simulink model "gate_V26_2016a"  (R2016a)
settings: Solver=FixedStepDiscrete  StartTime=0.0  StopTime=100  FixedStep=0.001  RelTol=1e-3
undefined symbols (not defined in the file or in its folder): CLOSE_CHAR, CLOSE_SIDE_VALUE, CLOSED, CLOSING, NO_PASS_ASSIG, OPEN, OPEN_CHAR, OPEN_SIDE_VALUE, OPEN_TIMEOUT, OPENING, OPENING_ACTIVE, PASS_ASSIGNED, PASS_INCOMPLETE, PASS_TIMEOUT, PASSWORD_VERIFIED, sigbuilder_block, TIMEOUT, WRONG_PASSWORD
libraries: simulink x9, arduinolib x5
(part 1 of 3)
settings Model: ExtModeTrigDuration=2  Creator=omaro  LastModifiedBy=omaro
settings OptimizationCC: StateBitsets=on  DataBitsets=on  LifeSpan=1  MaxStackSize=64
settings DebuggingCC: ConsistencyChecking=error  ArrayBoundsChecking=error  SignalInfNanChecking=error  SignalRangeChecking=error  ReadBeforeWriteMsg=EnableAllAsError  WriteAfterWriteMsg=EnableAllAsError  WriteAfterReadMsg=EnableAllAsError  AlgebraicLoopMsg=error  ArtificialAlgebraicLoopMsg=error  BlockPriorityViolationMsg=error  MinStepSizeMsg=error  CheckMatrixSingularityMsg=error  ParameterUnderflowMsg=error  ParameterPrecisionLossMsg=error  UnderSpecifiedDataTypeMsg=warning  UnnecessaryDatatypeConvMsg=warning  VectorMatrixConversionMsg=error  SignalLabelMismatchMsg=error  UnconnectedInputMsg=error  UnconnectedOutputMsg=error  UnconnectedLineMsg=error  SFcnCompatibilityMsg=warning  UniqueDataStoreMsg=error  BusObjectLabelMismatch=error  RootOutportRequireBusObject=error  ModelReferenceIOMsg=error  ModelReferenceVersionMismatchMessage=error  ModelReferenceIOMismatchMessage=error  ModelReferenceDataLoggingMessage=error  StrictBusMsg=ErrorOnBusTreatedAsVector  SFUnusedDataAndEventsDiag=error  SFUnexpectedBacktrackingDiag=error  SFInvalidInputDataAccessInChartInitDiag=error  SFNoUnconditionalDefaultTransitionDiag=error  SFTransitionOutsideNaturalParentDiag=error  SFUndirectedBroadcastEventsDiag=error  SFTransitionActionBeforeConditionDiag=error  SFOutputUsedAsStateInMooreChartDiag=warning
settings HardwareCC: ProdBitPerInt=16  ProdBitPerPointer=16  ProdLargestAtomicFloat=None  ProdWordSize=8  ProdHWDeviceType=Atmel->AVR
settings SFSimCC: SimCustomHeaderCode=|
  | //#include "C:\Users\omaro\Desktop\Gate_Model\Arduino\Arduino.h"
  | //#include "Keypad\Keypad.h"
settings RTWCC: SystemTargetFile=ert.tlc  HardwareBoard=Arduino Nano 3.0  TemplateMakefile=ert_default_tmf  GenerateReport=on  RTWUseSimCustomCode=on  Toolchain=Arduino AVR v1.6.1  BuildConfiguration=Faster Runs  LaunchReport=on
settings RTWCC: CustomHeaderCode=|
  | //#include "C:\Users\omaro\Desktop\Gate_Model\Arduino\Arduino.h"
  | //#include "Keypad\Keypad.h"
settings CodeAppCC: ForceParamTrailComments=on  OperatorAnnotations=on  MATLABSourceComments=on
settings ERTTargetCC: ERTCustomFileBanners=off  SupportContinuousTime=on  SupportNonInlinedSFcns=on  SupportVariableSizeSignals=on  ModelStepFunctionPrototypeControlCompliant=off  RootIOFormat=Structure reference

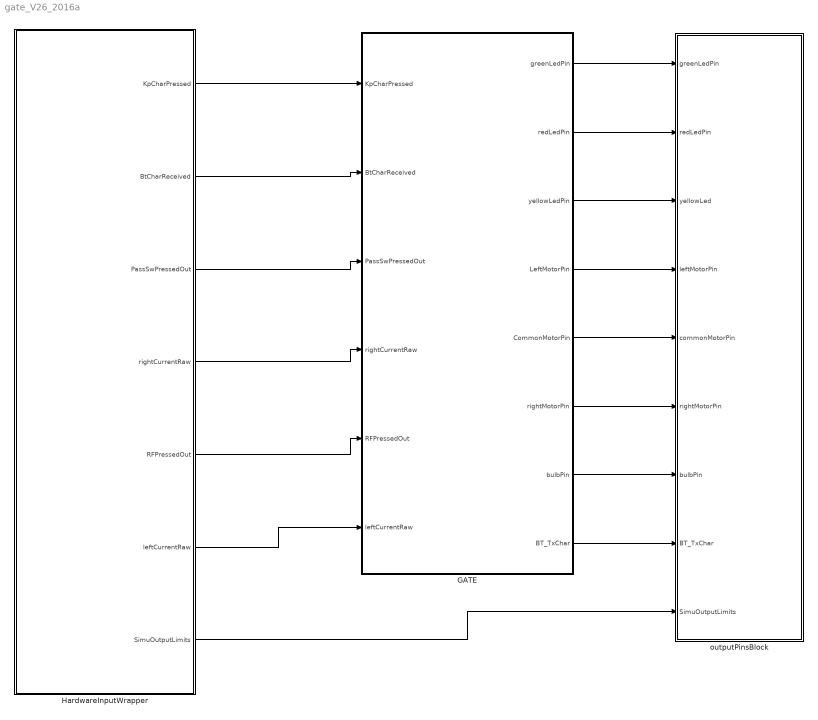
== system gate_V26_2016a ==
  GATE : Subsystem  Variant=on  VariantControl=Variant1  OverrideUsingVariant=Variant2
  HardwareInputWrapper : Subsystem  Variant=on  VariantControl=Variant1  OverrideUsingVariant=Variant2
  outputPinsBlock : Subsystem  Variant=on  VariantControl=Variant1  OverrideUsingVariant=Variant
  wires:
  HardwareInputWrapper/7(SimuOutputLimits) -> outputPinsBlock/9(SimuOutputLimits)
  HardwareInputWrapper/1(KpCharPressed) -> GATE/1("KpCharPressed ")
  HardwareInputWrapper/2(BtCharReceived) -> GATE/2("BtCharReceived ")
  HardwareInputWrapper/3(PassSwPressedOut) -> GATE/3("PassSwPressedOut ")
  HardwareInputWrapper/4(rightCurrentRaw) -> GATE/4(rightCurrentRaw)
  HardwareInputWrapper/5(RFPressedOut) -> GATE/5("RFPressedOut ")
  GATE/1(" greenLedPin") -> outputPinsBlock/1(greenLedPin)
  GATE/2(" redLedPin") -> outputPinsBlock/2(redLedPin)
  GATE/3(" yellowLedPin") -> outputPinsBlock/3(yellowLed)
  GATE/4(" LeftMotorPin") -> outputPinsBlock/4(leftMotorPin)
  GATE/5(" CommonMotorPin") -> outputPinsBlock/5(commonMotorPin)
  GATE/6(" rightMotorPin") -> outputPinsBlock/6(rightMotorPin)
  GATE/7(" bulbPin") -> outputPinsBlock/7(bulbPin)
  GATE/8(" BT_TxChar") -> outputPinsBlock/8(BT_TxChar)
  HardwareInputWrapper/6(leftCurrentRaw) -> GATE/6(leftCurrentRaw)

== system gate_V26_2016a/GATE ==
  "KpCharPressed " : Inport
  "BtCharReceived " : Inport  Port=2
  "PassSwPressedOut " : Inport  Port=3
  rightCurrentRaw : Inport  Port=4
  "RFPressedOut " : Inport  Port=5
  leftCurrentRaw : Inport  Port=6
  GATE_A : Subsystem  VariantControl=Variant1
  GATE_B : Subsystem  VariantControl=Variant2
  GATE_C : Subsystem  VariantControl=Variant3
  " greenLedPin" : Outport
  " redLedPin" : Outport  Port=2
  " yellowLedPin" : Outport  Port=3
  " LeftMotorPin" : Outport  Port=4
  " CommonMotorPin" : Outport  Port=5
  " rightMotorPin" : Outport  Port=6
  " bulbPin" : Outport  Port=7
  " BT_TxChar" : Outport  Port=8

== system gate_V26_2016a/HardwareInputWrapper ==
  HIL : Subsystem  VariantControl=Variant2
  MIL : Subsystem  VariantControl=Variant
  KpCharPressed : Outport
  BtCharReceived : Outport  Port=2
  PassSwPressedOut : Outport  Port=3
  rightCurrentRaw : Outport  Port=4
  RFPressedOut : Outport  Port=5
  leftCurrentRaw : Outport  Port=6
  SimuOutputLimits : Outport  Port=7

== system gate_V26_2016a/outputPinsBlock ==
  greenLedPin : Inport
  redLedPin : Inport  Port=2
  yellowLed : Inport  Port=3
  leftMotorPin : Inport  Port=4
  commonMotorPin : Inport  Port=5
  rightMotorPin : Inport  Port=6
  bulbPin : Inport  Port=7
  BT_TxChar : Inport  Port=8
  SimuOutputLimits : Inport  Port=9
  HIL : Subsystem  VariantControl=Variant
  MIL : Subsystem  Variant=on  VariantControl=Variant1  OverrideUsingVariant=Variant1

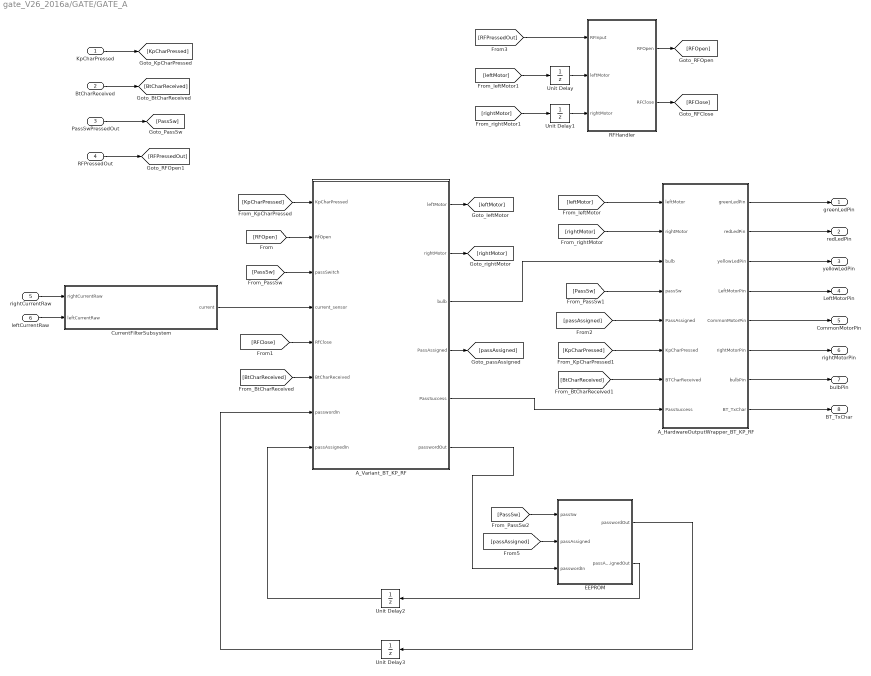
== system gate_V26_2016a/GATE/GATE_A ==
  KpCharPressed : Inport
  BtCharReceived : Inport  Port=2
  PassSwPressedOut : Inport  Port=3
  RFPressedOut : Inport  Port=4
  rightCurrentRaw : Inport  Port=5
  leftCurrentRaw : Inport  Port=6
  A_HardwareOutputWrapper_BT_KP_RF : Subsystem  VariantControl=Variant1
  A_Variant_BT_KP_RF : Subsystem  VariantControl=Variant
  CurrentFilterSubsystem : Subsystem
  EEPROM : Subsystem
  RFHandler : Subsystem
  Unit Delay{,1..3} (4 alike) : UnitDelay  SampleTime=-1
  greenLedPin : Outport
  redLedPin : Outport  Port=2
  yellowLedPin : Outport  Port=3
  LeftMotorPin : Outport  Port=4
  CommonMotorPin : Outport  Port=5
  rightMotorPin : Outport  Port=6
  bulbPin : Outport  Port=7
  BT_TxChar : Outport  Port=8
  wires:
  RFHandler/1(RFOpen) -> [RFOpen]
  RFHandler/2(RFClose) -> [RFClose]
  [RFPressedOut] -> RFHandler/1(RFInput)
  RFPressedOut/1 -> [RFPressedOut]
  PassSwPressedOut/1 -> [PassSw]
  [leftMotor] -> Unit Delay/1
  Unit Delay/1 -> RFHandler/2(leftMotor)
  [rightMotor] -> Unit Delay1/1
  Unit Delay1/1 -> RFHandler/3(rightMotor)
  BtCharReceived/1 -> [BtCharReceived]
  KpCharPressed/1 -> [KpCharPressed]
  [RFOpen] -> A_Variant_BT_KP_RF/2(RfOpen)
  [PassSw] -> A_Variant_BT_KP_RF/3(passSwitch)
  [RFClose] -> A_Variant_BT_KP_RF/5(RfClose)
  [BtCharReceived] -> A_Variant_BT_KP_RF/6(BtCharReceived)
  A_Variant_BT_KP_RF/1(leftMotor) -> [leftMotor]
  A_Variant_BT_KP_RF/2(rightMotor) -> [rightMotor]
  [KpCharPressed] -> A_Variant_BT_KP_RF/1(KpCharPressed)
  [leftMotor] -> A_HardwareOutputWrapper_BT_KP_RF/1(leftMotor)
  [rightMotor] -> A_HardwareOutputWrapper_BT_KP_RF/2(rightMotor)
  A_Variant_BT_KP_RF/3(bulb) -> A_HardwareOutputWrapper_BT_KP_RF/3(bulb)
  [PassSw] -> A_HardwareOutputWrapper_BT_KP_RF/4(passSw)
  [KpCharPressed] -> A_HardwareOutputWrapper_BT_KP_RF/6(KpCharPressed)
  [BtCharReceived] -> A_HardwareOutputWrapper_BT_KP_RF/7(BTCharReceived)
  A_HardwareOutputWrapper_BT_KP_RF/1(greenLedPin) -> greenLedPin/1
  A_HardwareOutputWrapper_BT_KP_RF/2(redLedPin) -> redLedPin/1
  A_HardwareOutputWrapper_BT_KP_RF/3(yellowLedPin) -> yellowLedPin/1
  A_HardwareOutputWrapper_BT_KP_RF/4(LeftMotorPin) -> LeftMotorPin/1
  A_HardwareOutputWrapper_BT_KP_RF/5(CommonMotorPin) -> CommonMotorPin/1
  A_HardwareOutputWrapper_BT_KP_RF/6(rightMotorPin) -> rightMotorPin/1
  A_HardwareOutputWrapper_BT_KP_RF/7(bulbPin) -> bulbPin/1
  A_HardwareOutputWrapper_BT_KP_RF/8(BT_TxChar) -> BT_TxChar/1
  A_Variant_BT_KP_RF/4(PassAssigned) -> [passAssigned]
  [passAssigned] -> A_HardwareOutputWrapper_BT_KP_RF/5(PassAssigned)
  [passAssigned] -> EEPROM/2(passAssigned)
  [PassSw] -> EEPROM/1(passSw)
  A_Variant_BT_KP_RF/6(passwordOut) -> EEPROM/3(passwordIn)
  EEPROM/1(passwordOut) -> Unit Delay3/1
  EEPROM/2(passAssignedOut) -> Unit Delay2/1
  Unit Delay2/1 -> A_Variant_BT_KP_RF/8(passAssignedIn)
  Unit Delay3/1 -> A_Variant_BT_KP_RF/7(passwordIn)
  A_Variant_BT_KP_RF/5(PassSuccess) -> A_HardwareOutputWrapper_BT_KP_RF/8(PassSuccess)
  CurrentFilterSubsystem/1(current) -> A_Variant_BT_KP_RF/4(current_sensor)
  rightCurrentRaw/1 -> CurrentFilterSubsystem/1(rightCurrentRaw)
  leftCurrentRaw/1 -> CurrentFilterSubsystem/2(leftCurrentRaw)

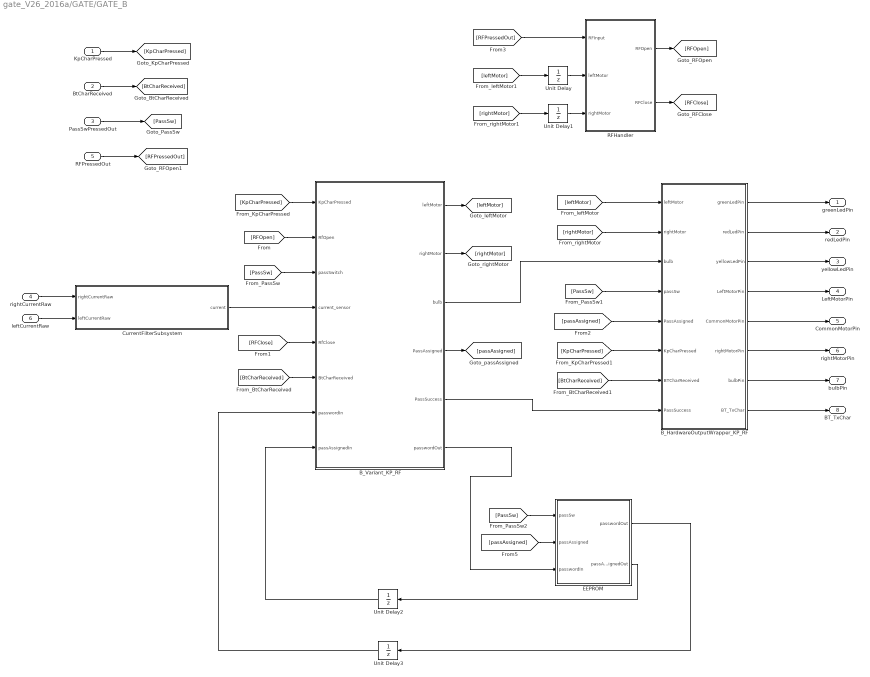
== system gate_V26_2016a/GATE/GATE_B ==
  KpCharPressed : Inport
  BtCharReceived : Inport  Port=2
  PassSwPressedOut : Inport  Port=3
  rightCurrentRaw : Inport  Port=4
  RFPressedOut : Inport  Port=5
  leftCurrentRaw : Inport  Port=6
  B_HardwareOutputWrapper_KP_RF : Subsystem  VariantControl=Variant2
  B_Variant_KP_RF : Subsystem  VariantControl=Variant2
  CurrentFilterSubsystem : Subsystem
  EEPROM : Subsystem
  RFHandler : Subsystem
  Unit Delay{,1..3} (4 alike) : UnitDelay  SampleTime=-1
  greenLedPin : Outport
  redLedPin : Outport  Port=2
  yellowLedPin : Outport  Port=3
  LeftMotorPin : Outport  Port=4
  CommonMotorPin : Outport  Port=5
  rightMotorPin : Outport  Port=6
  bulbPin : Outport  Port=7
  BT_TxChar : Outport  Port=8
  wires:
  CurrentFilterSubsystem/1(current) -> B_Variant_KP_RF/4(current_sensor)
  B_Variant_KP_RF/5(PassSuccess) -> B_HardwareOutputWrapper_KP_RF/8(PassSuccess)
  Unit Delay3/1 -> B_Variant_KP_RF/7(passwordIn)
  Unit Delay2/1 -> B_Variant_KP_RF/8(passAssignedIn)
  EEPROM/2(passAssignedOut) -> Unit Delay2/1
  EEPROM/1(passwordOut) -> Unit Delay3/1
  B_Variant_KP_RF/6(passwordOut) -> EEPROM/3(passwordIn)
  [PassSw] -> EEPROM/1(passSw)
  [passAssigned] -> EEPROM/2(passAssigned)
  [passAssigned] -> B_HardwareOutputWrapper_KP_RF/5(PassAssigned)
  B_Variant_KP_RF/4(PassAssigned) -> [passAssigned]
  B_HardwareOutputWrapper_KP_RF/8(BT_TxChar) -> BT_TxChar/1
  B_HardwareOutputWrapper_KP_RF/7(bulbPin) -> bulbPin/1
  B_HardwareOutputWrapper_KP_RF/6(rightMotorPin) -> rightMotorPin/1
  B_HardwareOutputWrapper_KP_RF/5(CommonMotorPin) -> CommonMotorPin/1
  B_HardwareOutputWrapper_KP_RF/4(LeftMotorPin) -> LeftMotorPin/1
  B_HardwareOutputWrapper_KP_RF/3(yellowLedPin) -> yellowLedPin/1
  B_HardwareOutputWrapper_KP_RF/2(redLedPin) -> redLedPin/1
  B_HardwareOutputWrapper_KP_RF/1(greenLedPin) -> greenLedPin/1
  [BtCharReceived] -> B_HardwareOutputWrapper_KP_RF/7(BTCharReceived)
  [KpCharPressed] -> B_HardwareOutputWrapper_KP_RF/6(KpCharPressed)
  [PassSw] -> B_HardwareOutputWrapper_KP_RF/4(passSw)
  B_Variant_KP_RF/3(bulb) -> B_HardwareOutputWrapper_KP_RF/3(bulb)
  [rightMotor] -> B_HardwareOutputWrapper_KP_RF/2(rightMotor)
  [leftMotor] -> B_HardwareOutputWrapper_KP_RF/1(leftMotor)
  [KpCharPressed] -> B_Variant_KP_RF/1(KpCharPressed)
  B_Variant_KP_RF/2(rightMotor) -> [rightMotor]
  B_Variant_KP_RF/1(leftMotor) -> [leftMotor]
  [BtCharReceived] -> B_Variant_KP_RF/6(BtCharReceived)
  [RFClose] -> B_Variant_KP_RF/5(RfClose)
  rightCurrentRaw/1 -> CurrentFilterSubsystem/1(rightCurrentRaw)
  [PassSw] -> B_Variant_KP_RF/3(passSwitch)
  [RFOpen] -> B_Variant_KP_RF/2(RfOpen)
  KpCharPressed/1 -> [KpCharPressed]
  BtCharReceived/1 -> [BtCharReceived]
  Unit Delay1/1 -> RFHandler/3(rightMotor)
  [rightMotor] -> Unit Delay1/1
  Unit Delay/1 -> RFHandler/2(leftMotor)
  [leftMotor] -> Unit Delay/1
  PassSwPressedOut/1 -> [PassSw]
  RFPressedOut/1 -> [RFPressedOut]
  [RFPressedOut] -> RFHandler/1(RFInput)
  RFHandler/2(RFClose) -> [RFClose]
  RFHandler/1(RFOpen) -> [RFOpen]
  leftCurrentRaw/1 -> CurrentFilterSubsystem/2(leftCurrentRaw)

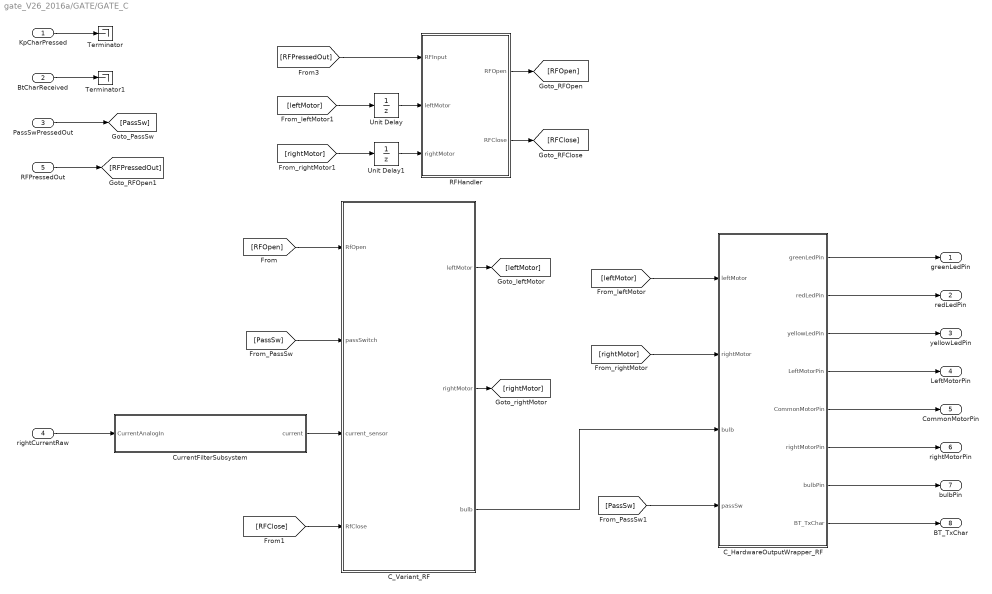
== system gate_V26_2016a/GATE/GATE_C ==
  KpCharPressed : Inport
  BtCharReceived : Inport  Port=2
  PassSwPressedOut : Inport  Port=3
  rightCurrentRaw : Inport  Port=4
  RFPressedOut : Inport  Port=5
  C_HardwareOutputWrapper_RF : Subsystem  VariantControl=Variant3
  C_Variant_RF : Subsystem  VariantControl=Variant3
  CurrentFilterSubsystem : Subsystem
  RFHandler : Subsystem
  Terminator : Terminator
  Terminator1 : Terminator
  Unit Delay : UnitDelay  SampleTime=-1
  Unit Delay1 : UnitDelay  SampleTime=-1
  greenLedPin : Outport
  redLedPin : Outport  Port=2
  yellowLedPin : Outport  Port=3
  LeftMotorPin : Outport  Port=4
  CommonMotorPin : Outport  Port=5
  rightMotorPin : Outport  Port=6
  bulbPin : Outport  Port=7
  BT_TxChar : Outport  Port=8
  wires:
  RFHandler/1(RFOpen) -> [RFOpen]
  RFHandler/2(RFClose) -> [RFClose]
  [RFPressedOut] -> RFHandler/1(RFInput)
  RFPressedOut/1 -> [RFPressedOut]
  PassSwPressedOut/1 -> [PassSw]
  [leftMotor] -> Unit Delay/1
  Unit Delay/1 -> RFHandler/2(leftMotor)
  [rightMotor] -> Unit Delay1/1
  Unit Delay1/1 -> RFHandler/3(rightMotor)
  BtCharReceived/1 -> Terminator1/1
  KpCharPressed/1 -> Terminator/1
  [RFOpen] -> C_Variant_RF/1(RfOpen)
  [PassSw] -> C_Variant_RF/2(passSwitch)
  rightCurrentRaw/1 -> CurrentFilterSubsystem/1(CurrentAnalogIn)
  [RFClose] -> C_Variant_RF/4(RfClose)
  C_Variant_RF/1(leftMotor) -> [leftMotor]
  C_Variant_RF/2(rightMotor) -> [rightMotor]
  [leftMotor] -> C_HardwareOutputWrapper_RF/1(leftMotor)
  [rightMotor] -> C_HardwareOutputWrapper_RF/2(rightMotor)
  C_Variant_RF/3(bulb) -> C_HardwareOutputWrapper_RF/3(bulb)
  [PassSw] -> C_HardwareOutputWrapper_RF/4(passSw)
  C_HardwareOutputWrapper_RF/1(greenLedPin) -> greenLedPin/1
  C_HardwareOutputWrapper_RF/2(redLedPin) -> redLedPin/1
  C_HardwareOutputWrapper_RF/3(yellowLedPin) -> yellowLedPin/1
  C_HardwareOutputWrapper_RF/4(LeftMotorPin) -> LeftMotorPin/1
  C_HardwareOutputWrapper_RF/5(CommonMotorPin) -> CommonMotorPin/1
  C_HardwareOutputWrapper_RF/6(rightMotorPin) -> rightMotorPin/1
  C_HardwareOutputWrapper_RF/7(bulbPin) -> bulbPin/1
  C_HardwareOutputWrapper_RF/8(BT_TxChar) -> BT_TxChar/1
  CurrentFilterSubsystem/1(current) -> C_Variant_RF/3(current_sensor)

== system gate_V26_2016a/HardwareInputWrapper/HIL ==
  Analog Input : arduinolib/Analog Input  pinNumber=6  sampleTime=-1  blockPlatform=arduino
  Analog Input1 : arduinolib/Analog Input  pinNumber=7  sampleTime=-1  blockPlatform=arduino
  BluetoothWrapper : Subsystem  Commented=on
  ButtonsPressed : Subsystem
  KeypadWrapper : Subsystem
  S-Function Builder1 : S-Function  Commented=on  InitFcn=try, set_param(gcb,'FunctionName','CurrentA_Lib'), end  FunctionName=CurrentA_Lib  SFunctionModules=CurrentA_Lib_wrapper  SFunctionDeploymentMode=off  EnableBusSupport=off  mask(S-Function Builder){}
      mask help: Simulink:masks:SFunctionBuilder_MD
      mask init:
      | val = [[.9  0.75 0.75 1 1 .9 .9 1]',[1 1 0.75 0.75 .9 .9 1 .9]'];try , sys = get_param(gcb,'SfunBuilderFcnName');if isempty(sys), sys = get_param(gcb,'FunctionName'); end,catch, sys = get_param(gcb,'FunctionName'); end
      settings: CopyFcn=set_param(gcbh,'LinkStatus','none')  PreSaveFcn=try, set_param(gcb,'FunctionName','CurrentA_Lib'), end  OpenFcn=sfunctionwizard(gcbh)
      mask Display: plot(val(:,1),val(:,2)),disp(sys), port_label('output',1,'currentValue')
  S-Function Builder2 : S-Function  Commented=on  InitFcn=try, set_param(gcb,'FunctionName','printingBlock'), end  FunctionName=printingBlock  SFunctionModules=printingBlock_wrapper  SFunctionDeploymentMode=off  EnableBusSupport=off  mask(S-Function Builder){}
      mask help: Simulink:masks:SFunctionBuilder_MD
      mask init: same as gate_V26_2016a/HardwareInputWrapper/HIL/S-Function Builder1
      settings: CopyFcn=set_param(gcbh,'LinkStatus','none')  PreSaveFcn=try, set_param(gcb,'FunctionName','printingBlock'), end  OpenFcn=sfunctionwizard(gcbh)
      mask Display: plot(val(:,1),val(:,2)),disp(sys), port_label('input',1,'uint8ToPrint')
  currentSensorWrapperOld : Subsystem  Commented=on
  KpCharPressed : Outport
  BtCharReceived : Outport  Port=2
  PassSwPressedOut : Outport  Port=3
  rightCurrentRaw : Outport  Port=4
  leftCurrentRaw : Outport  Port=5
  RFPressedOut : Outport  Port=6
  wires:
  BluetoothWrapper/1(bluetoothCharPressed) -> BtCharReceived/1
  Analog Input/1 -> rightCurrentRaw/1  "rightMotorSpeed"
  KeypadWrapper/1(charPressed) -> S-Function Builder2/1, KpCharPressed/1
  ButtonsPressed/2(SWPressed) -> PassSwPressedOut/1
  ButtonsPressed/1(RFPressed) -> RFPressedOut/1
  Analog Input1/1 -> leftCurrentRaw/1  "leftMotorSpeed"

== system gate_V26_2016a/HardwareInputWrapper/MIL ==
  Bus Creator : BusCreator  Inputs=16
  Quantizer{,1..3} (4 alike) : Quantizer  QuantizationInterval=-1
  Signal Builder : Subsystem  Tag=STV Subsys  LoadFcn=sigbuilder_block('load',[41.25 -234.75 971.25 378 ]);  StartFcn=sigbuilder_block('start');  StopFcn=sigbuilder_block('stop');  ClipboardFcn=sigbuilder_block('clipboard');  mask(Sigbuilder block){}
      mask help: Simulink:masks:SigbuilderBlock_MD
      mask init:
      | if ~strcmp(get_param(bdroot(gcbh),'SimulationStatus'),'stopped') tuvar = sigbuilder_block('maskInit'); end
      settings: CopyFcn=sigbuilder_block('copy');  DeleteFcn=sigbuilder_block('delete');  ModelCloseFcn=sigbuilder_block('modelClose');  PreSaveFcn=sigbuilder_block('preSave');  PauseFcn=sigbuilder_block('pause');  ContinueFcn=sigbuilder_block('continue');  NameChangeFcn=sigbuilder_block('namechange');  OpenFcn=sigbuilder_block('open',[6 28.2 1012.8 484.8 ]);  CloseFcn=sigbuilder_block('close');
      mask Display: plot(0, 0, 100, 100,[2, 2, 32, 32, 2], [68, 8, 8, 68, 68],[32, 2], [38, 38], [32, 19, 2],[53, 60, 44], [32, 17, 17, 2],[16, 16, 31, 31]);txt = getActiveGroup(gcbh);text(2, 100, txt,'verticalAlignment', 'top');
  KpCharPressed : Outport
  BtCharReceived : Outport  Port=2
  PassSwPressedOut : Outport  Port=3
  RFPressedOut : Outport  Port=4
  rightCurrentRaw : Outport  Port=5
  leftCurrentRaw : Outport  Port=6
  SimuOutputLimits : Outport  Port=7
  wires:
  Signal Builder/2(BT_input) -> Quantizer1/1
  Signal Builder/4(SW_input) -> Quantizer3/1
  Signal Builder/1(Kp_input) -> Quantizer/1
  Signal Builder/3(RF_input) -> Quantizer2/1
  Quantizer/1 -> KpCharPressed/1
  Quantizer1/1 -> BtCharReceived/1
  Quantizer2/1 -> RFPressedOut/1
  Quantizer3/1 -> PassSwPressedOut/1
  Bus Creator/1 -> SimuOutputLimits/1
  Signal Builder/17(GreenLedMax) -> Bus Creator/11  "GreenLedMax"
  Signal Builder/16(YellowLedMin) -> Bus Creator/10  "YellowLedMin"
  Signal Builder/18(GreenLedMin) -> Bus Creator/12  "GreenLedMin"
  Signal Builder/15(YellowLedMax) -> Bus Creator/9  "YellowLedMax"
  Signal Builder/19(BulbMax) -> Bus Creator/13  "BulbMax"
  Signal Builder/14(RedLedMin) -> Bus Creator/8  "RedLedMin"
  Signal Builder/20(BulbMin) -> Bus Creator/14  "BulbMin"
  Signal Builder/21(BT_outputMax) -> Bus Creator/15  "BT_outputMax"
  Signal Builder/13(RedLedMax) -> Bus Creator/7  "RedLedMax"
  Signal Builder/12(MCMin) -> Bus Creator/6  "MCMin"
  Signal Builder/11(MCMax) -> Bus Creator/5  "MCMax"
  Signal Builder/10(MRMin) -> Bus Creator/4  "MRMin"
  Signal Builder/9(MRMax) -> Bus Creator/3  "MRMax"
  Signal Builder/8(MLMin) -> Bus Creator/2  "MLMin"
  Signal Builder/7(MLMax) -> Bus Creator/1  "MLMax"
  Signal Builder/22(BT_outputMin) -> Bus Creator/16  "BT_outputMin"
  Signal Builder/5(rightSpeedRaw) -> rightCurrentRaw/1
  Signal Builder/6(leftSpeedRaw) -> leftCurrentRaw/1

== system gate_V26_2016a/outputPinsBlock/HIL ==
  greenLedPin : Inport
  redLedPin : Inport  Port=2
  yellowLed : Inport  Port=3
  leftMotorPin : Inport  Port=4
  commonMotorPin : Inport  Port=5
  rightMotorPin : Inport  Port=6
  bulbPin : Inport  Port=7
  Digital Output : arduinolib/Digital Output  pinNumber=11  blockPlatform=arduino
  Digital Output1 : arduinolib/Digital Output  pinNumber=12  blockPlatform=arduino
  Digital Output2 : arduinolib/Digital Output  pinNumber=13  blockPlatform=arduino
  S-Function Builder1 : S-Function  InitFcn=try, set_param(gcb,'FunctionName','A2PIN_Lib'), end  FunctionName=A2PIN_Lib  SFunctionModules=A2PIN_Lib_wrapper  SFunctionDeploymentMode=off  EnableBusSupport=off  mask(S-Function Builder){}
      mask help: Simulink:masks:SFunctionBuilder_MD
      mask init: same as gate_V26_2016a/HardwareInputWrapper/HIL/S-Function Builder1
      settings: CopyFcn=set_param(gcbh,'LinkStatus','none')  PreSaveFcn=try, set_param(gcb,'FunctionName','A2PIN_Lib'), end  OpenFcn=sfunctionwizard(gcbh)
      mask Display: plot(val(:,1),val(:,2)),disp(sys), port_label('input',1,'input')
  S-Function Builder2 : S-Function  InitFcn=try, set_param(gcb,'FunctionName','A3PIN_Lib'), end  FunctionName=A3PIN_Lib  SFunctionModules=A3PIN_Lib_wrapper  SFunctionDeploymentMode=off  EnableBusSupport=off  mask(S-Function Builder){}
      mask help: Simulink:masks:SFunctionBuilder_MD
      mask init: same as gate_V26_2016a/HardwareInputWrapper/HIL/S-Function Builder1
      settings: CopyFcn=set_param(gcbh,'LinkStatus','none')  PreSaveFcn=try, set_param(gcb,'FunctionName','A3PIN_Lib'), end  OpenFcn=sfunctionwizard(gcbh)
      mask Display: plot(val(:,1),val(:,2)),disp(sys), port_label('input',1,'input')
  S-Function Builder3 : S-Function  InitFcn=try, set_param(gcb,'FunctionName','A4PIN_Lib'), end  FunctionName=A4PIN_Lib  SFunctionModules=A4PIN_Lib_wrapper  SFunctionDeploymentMode=off  EnableBusSupport=off  mask(S-Function Builder){}
      mask help: Simulink:masks:SFunctionBuilder_MD
      mask init: same as gate_V26_2016a/HardwareInputWrapper/HIL/S-Function Builder1
      settings: CopyFcn=set_param(gcbh,'LinkStatus','none')  PreSaveFcn=try, set_param(gcb,'FunctionName','A4PIN_Lib'), end  OpenFcn=sfunctionwizard(gcbh)
      mask Display: plot(val(:,1),val(:,2)),disp(sys), port_label('input',1,'input')
  S-Function Builder4 : S-Function  InitFcn=try, set_param(gcb,'FunctionName','A5PIN_Lib'), end  FunctionName=A5PIN_Lib  SFunctionModules=A5PIN_Lib_wrapper  SFunctionDeploymentMode=off  EnableBusSupport=off  mask(S-Function Builder){}
      mask help: Simulink:masks:SFunctionBuilder_MD
      mask init: same as gate_V26_2016a/HardwareInputWrapper/HIL/S-Function Builder1
      settings: CopyFcn=set_param(gcbh,'LinkStatus','none')  PreSaveFcn=try, set_param(gcb,'FunctionName','A5PIN_Lib'), end  OpenFcn=sfunctionwizard(gcbh)
      mask Display: plot(val(:,1),val(:,2)),disp(sys), port_label('input',1,'input')
  wires:
  yellowLed/1 -> Digital Output2/1
  redLedPin/1 -> Digital Output/1
  greenLedPin/1 -> Digital Output1/1
  commonMotorPin/1 -> S-Function Builder3/1
  leftMotorPin/1 -> S-Function Builder2/1
  rightMotorPin/1 -> S-Function Builder4/1
  bulbPin/1 -> S-Function Builder1/1

== system gate_V26_2016a/outputPinsBlock/MIL ==
  "leftMotorPin " : Inport
  "commonMotorPin " : Inport  Port=2
  "rightMotorPin " : Inport  Port=3
  greenLedPin : Inport  Port=4
  redLedPin : Inport  Port=5
  yellowLed : Inport  Port=6
  bulbPin : Inport  Port=7
  BT_TxChar : Inport  Port=8
  SimuOutputLimits : Inport  Port=9
  ScopeBlocks : Subsystem  VariantControl=Variant1
  "VerificationBlocks " : Subsystem  VariantControl=Variant2

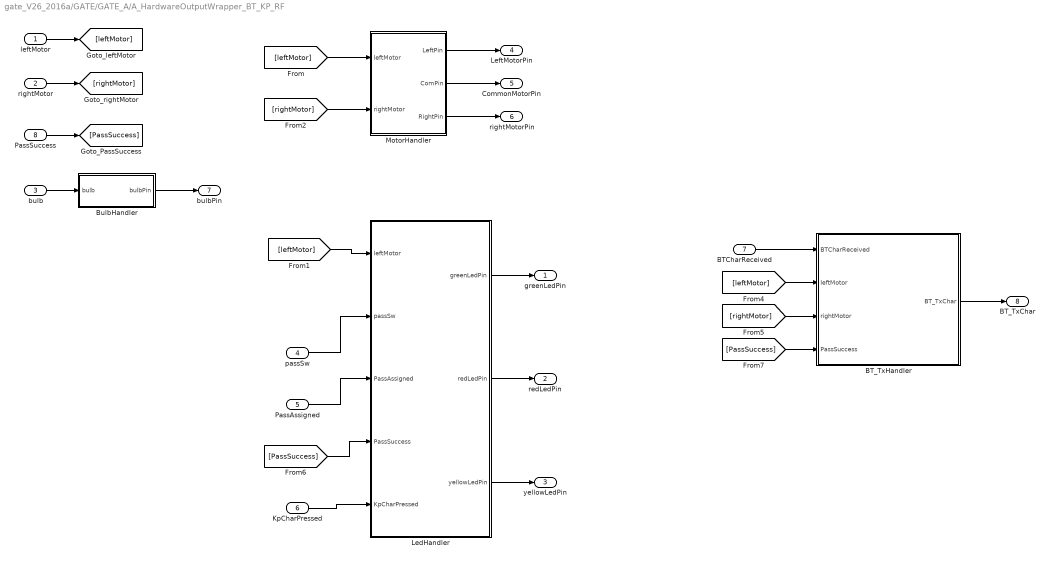
== system gate_V26_2016a/GATE/GATE_A/A_HardwareOutputWrapper_BT_KP_RF ==
  leftMotor : Inport
  rightMotor : Inport  Port=2
  bulb : Inport  Port=3
  passSw : Inport  Port=4
  PassAssigned : Inport  Port=5
  KpCharPressed : Inport  Port=6
  BTCharReceived : Inport  Port=7
  PassSuccess : Inport  Port=8
  BT_TxHandler : Subsystem
  BulbHandler : Subsystem
  LedHandler : Subsystem
  MotorHandler : Subsystem
  greenLedPin : Outport
  redLedPin : Outport  Port=2
  yellowLedPin : Outport  Port=3
  LeftMotorPin : Outport  Port=4
  CommonMotorPin : Outport  Port=5
  rightMotorPin : Outport  Port=6
  bulbPin : Outport  Port=7
  BT_TxChar : Outport  Port=8
  wires:
  [leftMotor] -> MotorHandler/1(leftMotor)
  [rightMotor] -> MotorHandler/2(rightMotor)
  bulb/1 -> BulbHandler/1(bulb)
  LedHandler/1(greenLedPin) -> greenLedPin/1
  LedHandler/2(redLedPin) -> redLedPin/1
  LedHandler/3(yellowLedPin) -> yellowLedPin/1
  MotorHandler/1(LeftPin) -> LeftMotorPin/1
  MotorHandler/2(ComPin) -> CommonMotorPin/1
  MotorHandler/3(RightPin) -> rightMotorPin/1
  BulbHandler/1(bulbPin) -> bulbPin/1
  leftMotor/1 -> [leftMotor]
  [leftMotor] -> LedHandler/1(leftMotor)
  rightMotor/1 -> [rightMotor]
  passSw/1 -> LedHandler/2(passSw)
  PassAssigned/1 -> LedHandler/3(PassAssigned)
  [PassSuccess] -> LedHandler/4(PassSuccess)
  KpCharPressed/1 -> LedHandler/5(KpCharPressed)
  [leftMotor] -> BT_TxHandler/2(leftMotor)
  BTCharReceived/1 -> BT_TxHandler/1(BTCharReceived)
  [rightMotor] -> BT_TxHandler/3(rightMotor)
  PassSuccess/1 -> [PassSuccess]
  [PassSuccess] -> BT_TxHandler/4(PassSuccess)
  BT_TxHandler/1(BT_TxChar) -> BT_TxChar/1

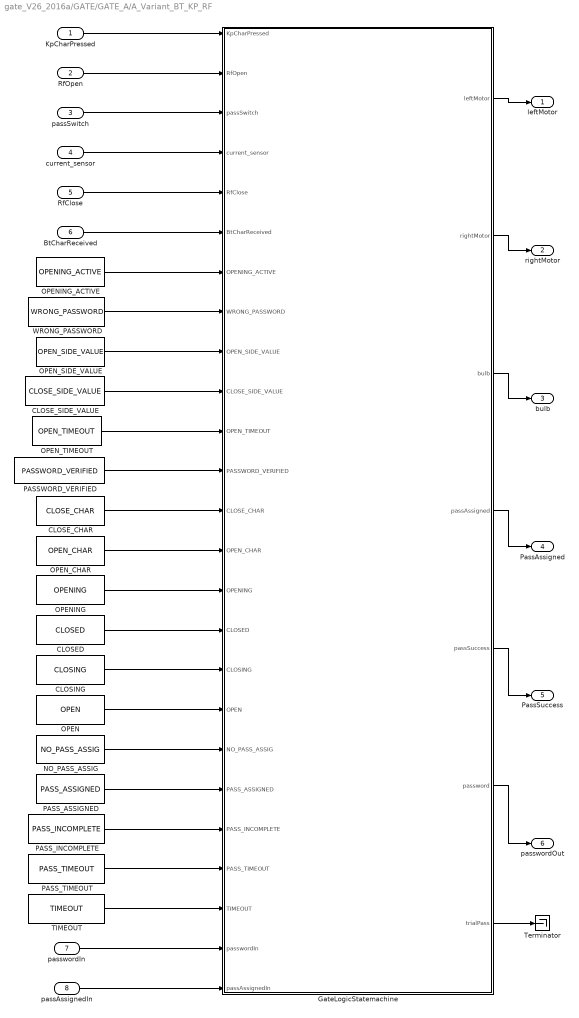
== system gate_V26_2016a/GATE/GATE_A/A_Variant_BT_KP_RF ==
  KpCharPressed : Inport
  RfOpen : Inport  Port=2
  passSwitch : Inport  Port=3
  current_sensor : Inport  Port=4
  RfClose : Inport  Port=5
  BtCharReceived : Inport  Port=6
  passwordIn : Inport  Port=7
  passAssignedIn : Inport  Port=8
  CLOSED : Constant  Value=CLOSED  SampleTime=-1
  CLOSE_CHAR : Constant  Value=CLOSE_CHAR  SampleTime=-1
  CLOSE_SIDE_VALUE : Constant  Value=CLOSE_SIDE_VALUE  SampleTime=-1
  CLOSING : Constant  Value=CLOSING  SampleTime=-1
  GateLogicStatemachine : Stateflow chart  TreatAsAtomicUnit=on
  NO_PASS_ASSIG : Constant  Value=NO_PASS_ASSIG  SampleTime=-1
  OPEN : Constant  Value=OPEN  SampleTime=-1
  OPENING : Constant  Value=OPENING  SampleTime=-1
  OPENING_ACTIVE : Constant  Value=OPENING_ACTIVE  SampleTime=-1
  OPEN_CHAR : Constant  Value=OPEN_CHAR  SampleTime=-1
  OPEN_SIDE_VALUE : Constant  Value=OPEN_SIDE_VALUE  SampleTime=-1
  OPEN_TIMEOUT : Constant  Value=OPEN_TIMEOUT  SampleTime=-1
  PASSWORD_VERIFIED : Constant  Value=PASSWORD_VERIFIED  SampleTime=-1
  PASS_ASSIGNED : Constant  Value=PASS_ASSIGNED  SampleTime=-1
  PASS_INCOMPLETE : Constant  Value=PASS_INCOMPLETE  SampleTime=-1
  PASS_TIMEOUT : Constant  Value=PASS_TIMEOUT  SampleTime=-1
  TIMEOUT : Constant  Value=TIMEOUT  SampleTime=-1
  Terminator : Terminator
  WRONG_PASSWORD : Constant  Value=WRONG_PASSWORD  SampleTime=-1
  leftMotor : Outport
  rightMotor : Outport  Port=2
  bulb : Outport  Port=3
  PassAssigned : Outport  Port=4
  PassSuccess : Outport  Port=5
  passwordOut : Outport  Port=6
  wires:
  RfClose/1 -> GateLogicStatemachine/5(RfClose)
  TIMEOUT/1 -> GateLogicStatemachine/23(TIMEOUT)
  PASS_INCOMPLETE/1 -> GateLogicStatemachine/21(PASS_INCOMPLETE)
  PASS_ASSIGNED/1 -> GateLogicStatemachine/20(PASS_ASSIGNED)
  GateLogicStatemachine/4(passAssigned) -> PassAssigned/1
  passSwitch/1 -> GateLogicStatemachine/3(passSwitch)
  GateLogicStatemachine/5(passSuccess) -> PassSuccess/1
  PASS_TIMEOUT/1 -> GateLogicStatemachine/22(PASS_TIMEOUT)
  KpCharPressed/1 -> GateLogicStatemachine/1(KpCharPressed)
  BtCharReceived/1 -> GateLogicStatemachine/6(BtCharReceived)
  NO_PASS_ASSIG/1 -> GateLogicStatemachine/19(NO_PASS_ASSIG)
  CLOSE_SIDE_VALUE/1 -> GateLogicStatemachine/10(CLOSE_SIDE_VALUE)
  OPEN_TIMEOUT/1 -> GateLogicStatemachine/11(OPEN_TIMEOUT)
  OPEN_SIDE_VALUE/1 -> GateLogicStatemachine/9(OPEN_SIDE_VALUE)
  OPENING_ACTIVE/1 -> GateLogicStatemachine/7(OPENING_ACTIVE)
  GateLogicStatemachine/2(rightMotor) -> rightMotor/1
  GateLogicStatemachine/1(leftMotor) -> leftMotor/1
  WRONG_PASSWORD/1 -> GateLogicStatemachine/8(WRONG_PASSWORD)
  current_sensor/1 -> GateLogicStatemachine/4(current_sensor)
  GateLogicStatemachine/3(bulb) -> bulb/1
  RfOpen/1 -> GateLogicStatemachine/2(RfOpen)
  PASSWORD_VERIFIED/1 -> GateLogicStatemachine/12(PASSWORD_VERIFIED)
  OPEN/1 -> GateLogicStatemachine/18(OPEN)
  CLOSE_CHAR/1 -> GateLogicStatemachine/13(CLOSE_CHAR)
  OPEN_CHAR/1 -> GateLogicStatemachine/14(OPEN_CHAR)
  CLOSED/1 -> GateLogicStatemachine/16(CLOSED)
  OPENING/1 -> GateLogicStatemachine/15(OPENING)
  CLOSING/1 -> GateLogicStatemachine/17(CLOSING)
  GateLogicStatemachine/6(password) -> passwordOut/1
  passwordIn/1 -> GateLogicStatemachine/24(passwordIn)
  passAssignedIn/1 -> GateLogicStatemachine/25(passAssignedIn)
  GateLogicStatemachine/7(trialPass) -> Terminator/1

== system gate_V26_2016a/GATE/GATE_A/CurrentFilterSubsystem ==
  rightCurrentRaw : Inport
  leftCurrentRaw : Inport  Port=2
  10msSmapler : Stateflow chart  TreatAsAtomicUnit=on
  Subsystem : Subsystem
  current : Outport
  wires:
  10msSmapler/1(triggerOn()) -> Subsystem/Trigger
  Subsystem/1(current) -> current/1
  rightCurrentRaw/1 -> Subsystem/1(rightCurrentRaw)
  leftCurrentRaw/1 -> Subsystem/2(leftCurrentRaw)

== system gate_V26_2016a/GATE/GATE_A/EEPROM ==
  passSw : Inport
  passAssigned : Inport  Port=2
  passwordIn : Inport  Port=3
  EEPROM_Control : Stateflow chart  TreatAsAtomicUnit=on
  EEPROM_UPDATE : Subsystem  TreatAsAtomicUnit=on
  Terminator : Terminator
  Unit Delay : UnitDelay  SampleTime=-1
  Unit Delay1 : UnitDelay  SampleTime=-1
  passwordOut : Outport
  passAssignedOut : Outport  Port=2
  wires:
  passSw/1 -> EEPROM_Control/1(passSw)
  Unit Delay/1 -> EEPROM_Control/3(readComplete)
  Unit Delay1/1 -> EEPROM_Control/4(writeComplete)
  EEPROM_Control/1(clearReq) -> EEPROM_UPDATE/1(clearReq)
  EEPROM_Control/2(readReq) -> EEPROM_UPDATE/2(readReq)
  EEPROM_Control/3(writeReq) -> EEPROM_UPDATE/3(writeReq)
  passwordIn/1 -> EEPROM_UPDATE/4(passwordIn)
  [passAssigned] -> EEPROM_Control/2(passAssigned)
  [passAssigned] -> EEPROM_UPDATE/5(passAssignedIn)
  passAssigned/1 -> [passAssigned]
  EEPROM_UPDATE/1(readComplete) -> [readComplete]
  [readComplete] -> Unit Delay/1
  [writeComplete] -> Unit Delay1/1
  EEPROM_UPDATE/2(writeComplete) -> [writeComplete]
  EEPROM_UPDATE/4(passwordOut) -> passwordOut/1
  EEPROM_UPDATE/5(passAssignedOut) -> passAssignedOut/1
  EEPROM_UPDATE/3(clearComplete) -> Terminator/1

== system gate_V26_2016a/GATE/GATE_A/RFHandler ==
  RFInput : Inport
  leftMotor : Inport  Port=2
  rightMotor : Inport  Port=3
  CLOSED : Constant  Value=CLOSED  SampleTime=-1
  CLOSING : Constant  Value=CLOSING  SampleTime=-1
  OPEN : Constant  Value=OPEN  SampleTime=-1
  OPENING : Constant  Value=OPENING  SampleTime=-1
  RFHandlerL : Stateflow chart  TreatAsAtomicUnit=on
  Scope : Scope
  RFOpen : Outport
  RFClose : Outport  Port=2
  wires:
  RFInput/1 -> RFHandlerL/1(btn)
  RFHandlerL/1(RFClose) -> RFClose/1
  RFHandlerL/2(RFOpen) -> Scope/1, RFOpen/1
  OPEN/1 -> RFHandlerL/6(OPEN)
  CLOSING/1 -> RFHandlerL/5(CLOSING)
  CLOSED/1 -> RFHandlerL/4(CLOSED)
  OPENING/1 -> RFHandlerL/7(OPENING)
  leftMotor/1 -> RFHandlerL/2(leftMotor)
  rightMotor/1 -> RFHandlerL/3(rightMotor)

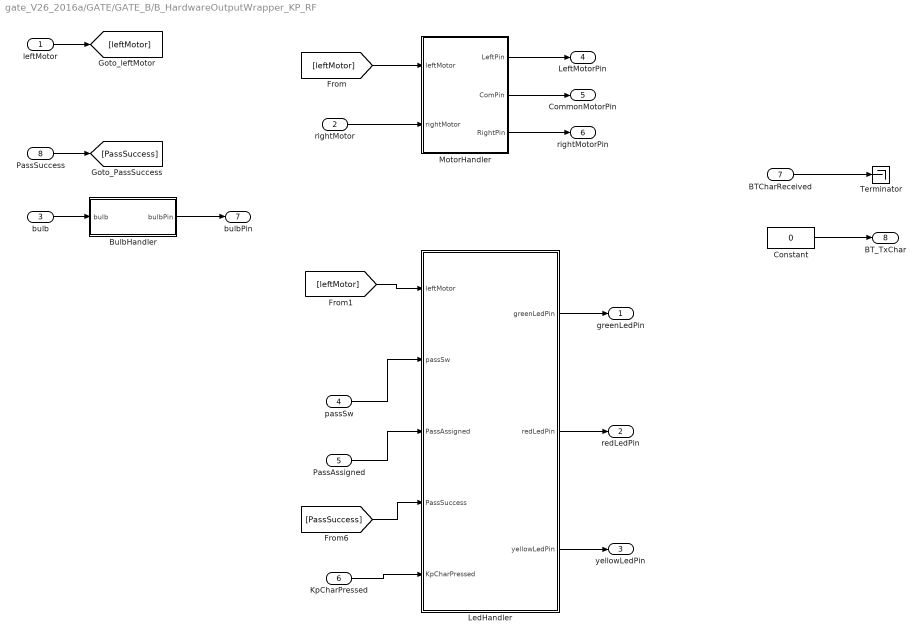
== system gate_V26_2016a/GATE/GATE_B/B_HardwareOutputWrapper_KP_RF ==
  leftMotor : Inport
  rightMotor : Inport  Port=2
  bulb : Inport  Port=3
  passSw : Inport  Port=4
  PassAssigned : Inport  Port=5
  KpCharPressed : Inport  Port=6
  BTCharReceived : Inport  Port=7
  PassSuccess : Inport  Port=8
  BulbHandler : Subsystem
  Constant : Constant  Value=0  SampleTime=-1
  LedHandler : Subsystem
  MotorHandler : Subsystem
  Terminator : Terminator
  greenLedPin : Outport
  redLedPin : Outport  Port=2
  yellowLedPin : Outport  Port=3
  LeftMotorPin : Outport  Port=4
  CommonMotorPin : Outport  Port=5
  rightMotorPin : Outport  Port=6
  bulbPin : Outport  Port=7
  BT_TxChar : Outport  Port=8
  wires:
  rightMotor/1 -> MotorHandler/2(rightMotor)
  BTCharReceived/1 -> Terminator/1
  [leftMotor] -> MotorHandler/1(leftMotor)
  bulb/1 -> BulbHandler/1(bulb)
  LedHandler/1(greenLedPin) -> greenLedPin/1
  LedHandler/2(redLedPin) -> redLedPin/1
  LedHandler/3(yellowLedPin) -> yellowLedPin/1
  MotorHandler/1(LeftPin) -> LeftMotorPin/1
  MotorHandler/2(ComPin) -> CommonMotorPin/1
  MotorHandler/3(RightPin) -> rightMotorPin/1
  BulbHandler/1(bulbPin) -> bulbPin/1
  leftMotor/1 -> [leftMotor]
  [leftMotor] -> LedHandler/1(leftMotor)
  passSw/1 -> LedHandler/2(passSw)
  PassAssigned/1 -> LedHandler/3(PassAssigned)
  [PassSuccess] -> LedHandler/4(PassSuccess)
  KpCharPressed/1 -> LedHandler/5(KpCharPressed)
  PassSuccess/1 -> [PassSuccess]
  Constant/1 -> BT_TxChar/1

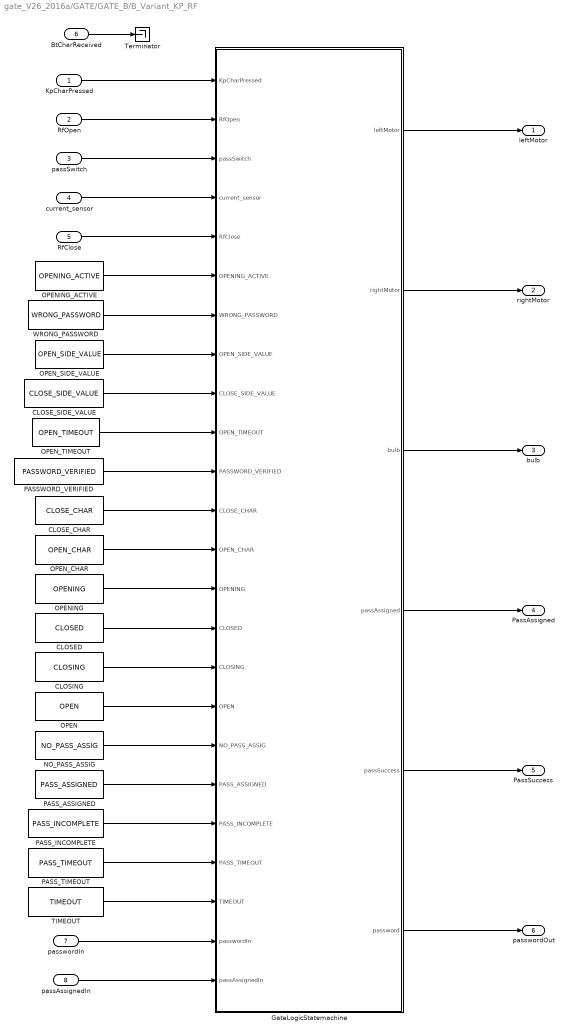
== system gate_V26_2016a/GATE/GATE_B/B_Variant_KP_RF ==
  KpCharPressed : Inport
  RfOpen : Inport  Port=2
  passSwitch : Inport  Port=3
  current_sensor : Inport  Port=4
  RfClose : Inport  Port=5
  BtCharReceived : Inport  Port=6
  passwordIn : Inport  Port=7
  passAssignedIn : Inport  Port=8
  CLOSED : Constant  Value=CLOSED  SampleTime=-1
  CLOSE_CHAR : Constant  Value=CLOSE_CHAR  SampleTime=-1
  CLOSE_SIDE_VALUE : Constant  Value=CLOSE_SIDE_VALUE  SampleTime=-1
  CLOSING : Constant  Value=CLOSING  SampleTime=-1
  GateLogicStatemachine : Stateflow chart  TreatAsAtomicUnit=on
  NO_PASS_ASSIG : Constant  Value=NO_PASS_ASSIG  SampleTime=-1
  OPEN : Constant  Value=OPEN  SampleTime=-1
  OPENING : Constant  Value=OPENING  SampleTime=-1
  OPENING_ACTIVE : Constant  Value=OPENING_ACTIVE  SampleTime=-1
  OPEN_CHAR : Constant  Value=OPEN_CHAR  SampleTime=-1
  OPEN_SIDE_VALUE : Constant  Value=OPEN_SIDE_VALUE  SampleTime=-1
  OPEN_TIMEOUT : Constant  Value=OPEN_TIMEOUT  SampleTime=-1
  PASSWORD_VERIFIED : Constant  Value=PASSWORD_VERIFIED  SampleTime=-1
  PASS_ASSIGNED : Constant  Value=PASS_ASSIGNED  SampleTime=-1
  PASS_INCOMPLETE : Constant  Value=PASS_INCOMPLETE  SampleTime=-1
  PASS_TIMEOUT : Constant  Value=PASS_TIMEOUT  SampleTime=-1
  TIMEOUT : Constant  Value=TIMEOUT  SampleTime=-1
  Terminator : Terminator
  WRONG_PASSWORD : Constant  Value=WRONG_PASSWORD  SampleTime=-1
  leftMotor : Outport
  rightMotor : Outport  Port=2
  bulb : Outport  Port=3
  PassAssigned : Outport  Port=4
  PassSuccess : Outport  Port=5
  passwordOut : Outport  Port=6
  wires:
  GateLogicStatemachine/6(password) -> passwordOut/1
  passAssignedIn/1 -> GateLogicStatemachine/24(passAssignedIn)
  passwordIn/1 -> GateLogicStatemachine/23(passwordIn)
  BtCharReceived/1 -> Terminator/1
  RfClose/1 -> GateLogicStatemachine/5(RfClose)
  TIMEOUT/1 -> GateLogicStatemachine/22(TIMEOUT)
  PASS_INCOMPLETE/1 -> GateLogicStatemachine/20(PASS_INCOMPLETE)
  PASS_ASSIGNED/1 -> GateLogicStatemachine/19(PASS_ASSIGNED)
  GateLogicStatemachine/4(passAssigned) -> PassAssigned/1
  passSwitch/1 -> GateLogicStatemachine/3(passSwitch)
  GateLogicStatemachine/5(passSuccess) -> PassSuccess/1
  PASS_TIMEOUT/1 -> GateLogicStatemachine/21(PASS_TIMEOUT)
  KpCharPressed/1 -> GateLogicStatemachine/1(KpCharPressed)
  NO_PASS_ASSIG/1 -> GateLogicStatemachine/18(NO_PASS_ASSIG)
  CLOSE_SIDE_VALUE/1 -> GateLogicStatemachine/9(CLOSE_SIDE_VALUE)
  OPEN_TIMEOUT/1 -> GateLogicStatemachine/10(OPEN_TIMEOUT)
  OPEN_SIDE_VALUE/1 -> GateLogicStatemachine/8(OPEN_SIDE_VALUE)
  OPENING_ACTIVE/1 -> GateLogicStatemachine/6(OPENING_ACTIVE)
  GateLogicStatemachine/2(rightMotor) -> rightMotor/1
  GateLogicStatemachine/1(leftMotor) -> leftMotor/1
  WRONG_PASSWORD/1 -> GateLogicStatemachine/7(WRONG_PASSWORD)
  current_sensor/1 -> GateLogicStatemachine/4(current_sensor)
  GateLogicStatemachine/3(bulb) -> bulb/1
  RfOpen/1 -> GateLogicStatemachine/2(RfOpen)
  PASSWORD_VERIFIED/1 -> GateLogicStatemachine/11(PASSWORD_VERIFIED)
  OPEN/1 -> GateLogicStatemachine/17(OPEN)
  CLOSE_CHAR/1 -> GateLogicStatemachine/12(CLOSE_CHAR)
  OPEN_CHAR/1 -> GateLogicStatemachine/13(OPEN_CHAR)
  CLOSED/1 -> GateLogicStatemachine/15(CLOSED)
  OPENING/1 -> GateLogicStatemachine/14(OPENING)
  CLOSING/1 -> GateLogicStatemachine/16(CLOSING)

== system gate_V26_2016a/GATE/GATE_B/CurrentFilterSubsystem ==
  rightCurrentRaw : Inport
  leftCurrentRaw : Inport  Port=2
  10msSmapler : Stateflow chart  TreatAsAtomicUnit=on
  Subsystem : Subsystem
  current : Outport
  wires:
  10msSmapler/1(triggerOn()) -> Subsystem/Trigger
  Subsystem/1(current) -> current/1
  rightCurrentRaw/1 -> Subsystem/1(rightCurrentRaw)
  leftCurrentRaw/1 -> Subsystem/2(leftCurrentRaw)

== system gate_V26_2016a/GATE/GATE_B/EEPROM ==
  passSw : Inport
  passAssigned : Inport  Port=2
  passwordIn : Inport  Port=3
  EEPROM_Control : Stateflow chart  TreatAsAtomicUnit=on
  EEPROM_UPDATE : Subsystem  TreatAsAtomicUnit=on
  Terminator : Terminator
  Unit Delay : UnitDelay  SampleTime=-1
  Unit Delay1 : UnitDelay  SampleTime=-1
  passwordOut : Outport
  passAssignedOut : Outport  Port=2
  wires:
  EEPROM_UPDATE/3(clearComplete) -> Terminator/1
  EEPROM_UPDATE/5(passAssignedOut) -> passAssignedOut/1
  EEPROM_UPDATE/4(passwordOut) -> passwordOut/1
  EEPROM_UPDATE/2(writeComplete) -> [writeComplete]
  [writeComplete] -> Unit Delay1/1
  [readComplete] -> Unit Delay/1
  EEPROM_UPDATE/1(readComplete) -> [readComplete]
  passAssigned/1 -> [passAssigned]
  [passAssigned] -> EEPROM_UPDATE/5(passAssignedIn)
  [passAssigned] -> EEPROM_Control/2(passAssigned)
  passwordIn/1 -> EEPROM_UPDATE/4(passwordIn)
  EEPROM_Control/3(writeReq) -> EEPROM_UPDATE/3(writeReq)
  EEPROM_Control/2(readReq) -> EEPROM_UPDATE/2(readReq)
  EEPROM_Control/1(clearReq) -> EEPROM_UPDATE/1(clearReq)
  Unit Delay1/1 -> EEPROM_Control/4(writeComplete)
  Unit Delay/1 -> EEPROM_Control/3(readComplete)
  passSw/1 -> EEPROM_Control/1(passSw)

== system gate_V26_2016a/GATE/GATE_B/RFHandler ==
  RFInput : Inport
  leftMotor : Inport  Port=2
  rightMotor : Inport  Port=3
  CLOSED : Constant  Value=CLOSED  SampleTime=-1
  CLOSING : Constant  Value=CLOSING  SampleTime=-1
  OPEN : Constant  Value=OPEN  SampleTime=-1
  OPENING : Constant  Value=OPENING  SampleTime=-1
  RFHandlerL : Stateflow chart  TreatAsAtomicUnit=on
  Scope : Scope
  RFOpen : Outport
  RFClose : Outport  Port=2
  wires:
  rightMotor/1 -> RFHandlerL/3(rightMotor)
  leftMotor/1 -> RFHandlerL/2(leftMotor)
  OPENING/1 -> RFHandlerL/7(OPENING)
  CLOSED/1 -> RFHandlerL/4(CLOSED)
  CLOSING/1 -> RFHandlerL/5(CLOSING)
  OPEN/1 -> RFHandlerL/6(OPEN)
  RFHandlerL/2(RFOpen) -> RFOpen/1, Scope/1
  RFHandlerL/1(RFClose) -> RFClose/1
  RFInput/1 -> RFHandlerL/1(btn)

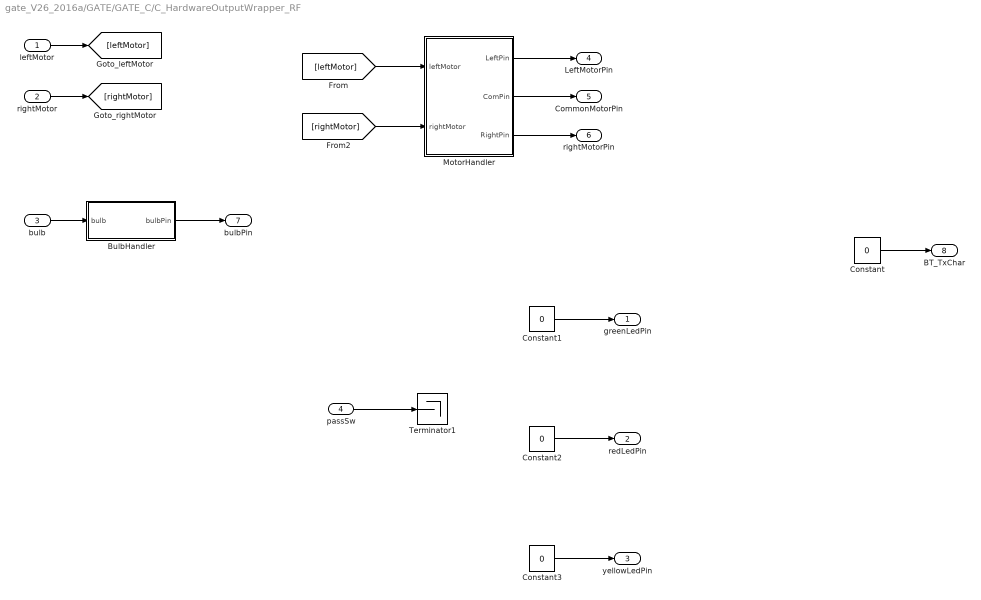
== system gate_V26_2016a/GATE/GATE_C/C_HardwareOutputWrapper_RF ==
  leftMotor : Inport
  rightMotor : Inport  Port=2
  bulb : Inport  Port=3
  passSw : Inport  Port=4
  BulbHandler : Subsystem
  Constant{,1..3} (4 alike) : Constant  Value=0  SampleTime=-1
  MotorHandler : Subsystem
  Terminator1 : Terminator
  greenLedPin : Outport
  redLedPin : Outport  Port=2
  yellowLedPin : Outport  Port=3
  LeftMotorPin : Outport  Port=4
  CommonMotorPin : Outport  Port=5
  rightMotorPin : Outport  Port=6
  bulbPin : Outport  Port=7
  BT_TxChar : Outport  Port=8
  wires:
  [leftMotor] -> MotorHandler/1(leftMotor)
  [rightMotor] -> MotorHandler/2(rightMotor)
  bulb/1 -> BulbHandler/1(bulb)
  MotorHandler/1(LeftPin) -> LeftMotorPin/1
  MotorHandler/2(ComPin) -> CommonMotorPin/1
  MotorHandler/3(RightPin) -> rightMotorPin/1
  BulbHandler/1(bulbPin) -> bulbPin/1
  leftMotor/1 -> [leftMotor]
  rightMotor/1 -> [rightMotor]
  Constant/1 -> BT_TxChar/1
  Constant3/1 -> yellowLedPin/1
  Constant2/1 -> redLedPin/1
  Constant1/1 -> greenLedPin/1
  passSw/1 -> Terminator1/1

== system gate_V26_2016a/GATE/GATE_C/C_Variant_RF ==
  RfOpen : Inport
  passSwitch : Inport  Port=2
  current_sensor : Inport  Port=3
  RfClose : Inport  Port=4
  CLOSED : Constant  Value=CLOSED  SampleTime=-1
  CLOSE_SIDE_VALUE : Constant  Value=CLOSE_SIDE_VALUE  SampleTime=-1
  CLOSING : Constant  Value=CLOSING  SampleTime=-1
  GateLogicStatemachine : Stateflow chart  TreatAsAtomicUnit=on
  OPEN : Constant  Value=OPEN  SampleTime=-1
  OPENING : Constant  Value=OPENING  SampleTime=-1
  OPENING_ACTIVE : Constant  Value=OPENING_ACTIVE  SampleTime=-1
  OPEN_SIDE_VALUE : Constant  Value=OPEN_SIDE_VALUE  SampleTime=-1
  OPEN_TIMEOUT : Constant  Value=OPEN_TIMEOUT  SampleTime=-1
  leftMotor : Outport
  rightMotor : Outport  Port=2
  bulb : Outport  Port=3
  wires:
  RfClose/1 -> GateLogicStatemachine/4(RfClose)
  passSwitch/1 -> GateLogicStatemachine/2(passSwitch)
  CLOSE_SIDE_VALUE/1 -> GateLogicStatemachine/7(CLOSE_SIDE_VALUE)
  OPEN_TIMEOUT/1 -> GateLogicStatemachine/8(OPEN_TIMEOUT)
  OPEN_SIDE_VALUE/1 -> GateLogicStatemachine/6(OPEN_SIDE_VALUE)
  OPENING_ACTIVE/1 -> GateLogicStatemachine/5(OPENING_ACTIVE)
  GateLogicStatemachine/2(rightMotor) -> rightMotor/1
  GateLogicStatemachine/1(leftMotor) -> leftMotor/1
  current_sensor/1 -> GateLogicStatemachine/3(current_sensor)
  GateLogicStatemachine/3(bulb) -> bulb/1
  RfOpen/1 -> GateLogicStatemachine/1(RfOpen)
  OPEN/1 -> GateLogicStatemachine/12(OPEN)
  CLOSED/1 -> GateLogicStatemachine/10(CLOSED)
  OPENING/1 -> GateLogicStatemachine/9(OPENING)
  CLOSING/1 -> GateLogicStatemachine/11(CLOSING)

== system gate_V26_2016a/GATE/GATE_C/CurrentFilterSubsystem ==
  CurrentAnalogIn : Inport
  10msSmapler : Stateflow chart  TreatAsAtomicUnit=on
  Subsystem : Subsystem
  current : Outport
  wires:
  CurrentAnalogIn/1 -> Subsystem/1(CurrentAnalogIn)
  Subsystem/1(current) -> current/1
  10msSmapler/1(triggerOn()) -> Subsystem/Trigger

== system gate_V26_2016a/GATE/GATE_C/RFHandler ==
  RFInput : Inport
  leftMotor : Inport  Port=2
  rightMotor : Inport  Port=3
  CLOSED : Constant  Value=CLOSED  SampleTime=-1
  CLOSING : Constant  Value=CLOSING  SampleTime=-1
  OPEN : Constant  Value=OPEN  SampleTime=-1
  OPENING : Constant  Value=OPENING  SampleTime=-1
  RFHandlerL : Stateflow chart  TreatAsAtomicUnit=on
  RFOpen : Outport
  RFClose : Outport  Port=2
  wires:
  RFInput/1 -> RFHandlerL/1(btn)
  RFHandlerL/1(RFClose) -> RFClose/1
  RFHandlerL/2(RFOpen) -> RFOpen/1
  OPEN/1 -> RFHandlerL/6(OPEN)
  CLOSING/1 -> RFHandlerL/5(CLOSING)
  CLOSED/1 -> RFHandlerL/4(CLOSED)
  OPENING/1 -> RFHandlerL/7(OPENING)
  leftMotor/1 -> RFHandlerL/2(leftMotor)
  rightMotor/1 -> RFHandlerL/3(rightMotor)

== system gate_V26_2016a/HardwareInputWrapper/HIL/BluetoothWrapper ==
  S-Function Builder : S-Function  InitFcn=try, set_param(gcb,'FunctionName','BluetoothLib'), end  FunctionName=BluetoothLib  SFunctionModules=BluetoothLib_wrapper  SFunctionDeploymentMode=off  EnableBusSupport=off  mask(S-Function Builder){}
      mask help: Simulink:masks:SFunctionBuilder_MD
      mask init: same as gate_V26_2016a/HardwareInputWrapper/HIL/S-Function Builder1
      settings: CopyFcn=set_param(gcbh,'LinkStatus','none')  PreSaveFcn=try, set_param(gcb,'FunctionName','BluetoothLib'), end  OpenFcn=sfunctionwizard(gcbh)
      mask Display: plot(val(:,1),val(:,2)),disp(sys), port_label('output',1,'BtCharRecieved')
  S-Function Builder1 : S-Function  Commented=on  InitFcn=try, set_param(gcb,'FunctionName','printingBlock'), end  FunctionName=printingBlock  SFunctionModules=printingBlock_wrapper  SFunctionDeploymentMode=off  EnableBusSupport=off  mask(S-Function Builder){}
      mask help: Simulink:masks:SFunctionBuilder_MD
      mask init: same as gate_V26_2016a/HardwareInputWrapper/HIL/S-Function Builder1
      settings: CopyFcn=set_param(gcbh,'LinkStatus','none')  PreSaveFcn=try, set_param(gcb,'FunctionName','printingBlock'), end  OpenFcn=sfunctionwizard(gcbh)
      mask Display: plot(val(:,1),val(:,2)),disp(sys), port_label('input',1,'input'), port_label('input',2,'oldInput')
  Unit Delay : UnitDelay  Commented=on  SampleTime=-1
  bluetoothCharPressed : Outport
  wires:
  S-Function Builder/1 -> S-Function Builder1/1, Unit Delay/1, bluetoothCharPressed/1
  Unit Delay/1 -> S-Function Builder1/2

== system gate_V26_2016a/HardwareInputWrapper/HIL/ButtonsPressed ==
  S-Function Builder1 : S-Function  InitFcn=try, set_param(gcb,'FunctionName','Button_Lib'), end  FunctionName=Button_Lib  SFunctionModules=Button_Lib_wrapper  SFunctionDeploymentMode=off  EnableBusSupport=off  mask(S-Function Builder){}
      mask help: Simulink:masks:SFunctionBuilder_MD
      mask init: same as gate_V26_2016a/HardwareInputWrapper/HIL/S-Function Builder1
      settings: CopyFcn=set_param(gcbh,'LinkStatus','none')  PreSaveFcn=try, set_param(gcb,'FunctionName','Button_Lib'), end  OpenFcn=sfunctionwizard(gcbh)
      mask Display: plot(val(:,1),val(:,2)),disp(sys), port_label('output',1,'RFInput'), port_label('output',2,'passSw')
  RFPressed : Outport
  SWPressed : Outport  Port=2
  wires:
  S-Function Builder1/1 -> RFPressed/1
  S-Function Builder1/2 -> SWPressed/1

== system gate_V26_2016a/HardwareInputWrapper/HIL/KeypadWrapper ==
  KeypadLib : S-Function  InitFcn=try, set_param(gcb,'FunctionName','keypadLib'), end  FunctionName=keypadLib  SFunctionModules=keypadLib_wrapper  SFunctionDeploymentMode=off  EnableBusSupport=off  mask(S-Function Builder){}
      mask help: Simulink:masks:SFunctionBuilder_MD
      mask init: same as gate_V26_2016a/HardwareInputWrapper/HIL/S-Function Builder1
      settings: CopyFcn=set_param(gcbh,'LinkStatus','none')  PreSaveFcn=try, set_param(gcb,'FunctionName','keypadLib'), end  OpenFcn=sfunctionwizard(gcbh)
      mask Display: plot(val(:,1),val(:,2)),disp(sys), port_label('output',1,'charPressed')
  charPressed : Outport
  wires:
  KeypadLib/1 -> charPressed/1

== system gate_V26_2016a/HardwareInputWrapper/HIL/currentSensorWrapperOld ==
  CurrentAnalogIn : Inport
  Add : Sum  Commented=on
  Constant : Constant  Commented=on  Value=0
  Constant1 : Constant  Commented=on
  Divide : Product  Commented=on  Inputs=*/
  Divide1 : Product  Commented=on  Inputs=*/
  MaxAnalog : Constant  Commented=on  Value=65535
  MaxAnalog1 : Constant  Commented=on
  MaxAnalog2 : Constant  Commented=on  Value=600
  MaxVoltage : Constant  Commented=on  Value=5
  Product : Product  Commented=on
  Relational Operator : RelationalOperator  Commented=on  Operator=<=  OutDataTypeStr=boolean
  Slider Gain : simulink/Math Operations/Slider Gain  Commented=on  low=0  gain=1  high=255
  SquareWaveDetector : Stateflow chart  TreatAsAtomicUnit=on
  Subtract : Sum  Commented=on  Inputs=+-
  Switch : Switch  Commented=on  Criteria=u2 > Threshold
  constantInCurrentEqua : Constant  Commented=on  Value=2.5
  constantInCurrentEqua1 : Constant  Commented=on  Value=0.2
  current : Outport
  wires:
  MaxAnalog/1 -> Divide/2
  Divide/1 -> Product/1
  MaxVoltage/1 -> Product/2
  Product/1 -> Subtract/1
  constantInCurrentEqua/1 -> Subtract/2
  Subtract/1 -> Divide1/1
  constantInCurrentEqua1/1 -> Divide1/2
  Slider Gain/1 -> Divide/1
  Add/1 -> Slider Gain/1
  MaxAnalog1/1 -> Add/1
  MaxAnalog2/1 -> Relational Operator/2
  Relational Operator/1 -> Switch/2
  Constant1/1 -> Switch/3
  Constant/1 -> Switch/1
  CurrentAnalogIn/1 -> SquareWaveDetector/1(CurrentAnalogIn)
  SquareWaveDetector/1(currentValue) -> current/1

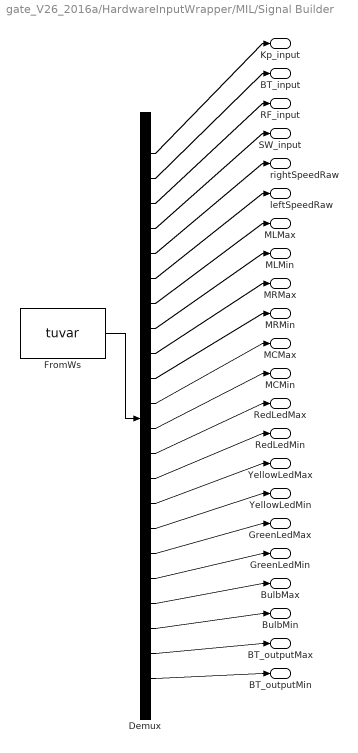
== system gate_V26_2016a/HardwareInputWrapper/MIL/Signal Builder ==
  Demux : Demux  Tag=STV Demux  Outputs=22
  FromWs : FromWorkspace  Tag=STV FromWs  VariableName=tuvar  SampleTime=0
  Kp_input : Outport  Tag=STV Outport
  BT_input : Outport  Tag=STV Outport  Port=2
  RF_input : Outport  Tag=STV Outport  Port=3
  SW_input : Outport  Tag=STV Outport  Port=4
  rightSpeedRaw : Outport  Tag=STV Outport  Port=5
  leftSpeedRaw : Outport  Tag=STV Outport  Port=6
  MLMax : Outport  Tag=STV Outport  Port=7
  MLMin : Outport  Tag=STV Outport  Port=8
  MRMax : Outport  Tag=STV Outport  Port=9
  MRMin : Outport  Tag=STV Outport  Port=10
  MCMax : Outport  Tag=STV Outport  Port=11
  MCMin : Outport  Tag=STV Outport  Port=12
  RedLedMax : Outport  Tag=STV Outport  Port=13
  RedLedMin : Outport  Tag=STV Outport  Port=14
  YellowLedMax : Outport  Tag=STV Outport  Port=15
  YellowLedMin : Outport  Tag=STV Outport  Port=16
  GreenLedMax : Outport  Tag=STV Outport  Port=17
  GreenLedMin : Outport  Tag=STV Outport  Port=18
  BulbMax : Outport  Tag=STV Outport  Port=19
  BulbMin : Outport  Tag=STV Outport  Port=20
  BT_outputMax : Outport  Tag=STV Outport  Port=21
  BT_outputMin : Outport  Tag=STV Outport  Port=22
  wires:
  FromWs/1 -> Demux/1
  Demux/1 -> Kp_input/1
  Demux/2 -> BT_input/1
  Demux/3 -> RF_input/1
  Demux/4 -> SW_input/1
  Demux/5 -> rightSpeedRaw/1
  Demux/6 -> leftSpeedRaw/1
  Demux/7 -> MLMax/1
  Demux/8 -> MLMin/1
  Demux/9 -> MRMax/1
  Demux/10 -> MRMin/1
  Demux/11 -> MCMax/1
  Demux/12 -> MCMin/1
  Demux/13 -> RedLedMax/1
  Demux/14 -> RedLedMin/1
  Demux/15 -> YellowLedMax/1
  Demux/16 -> YellowLedMin/1
  Demux/17 -> GreenLedMax/1
  Demux/18 -> GreenLedMin/1
  Demux/19 -> BulbMax/1
  Demux/20 -> BulbMin/1
  Demux/21 -> BT_outputMax/1
  Demux/22 -> BT_outputMin/1
